simulink model "Non_Linearizzato_LQG"  (R2024b)
settings: Solver=VariableStepAuto  StartTime=0.0  StopTime=30  RelTol=1e-3
values from neighbouring files (symbols this model uses):
  Anom = A.NominalValue    [Parameter_CSI.m]
  Bnom = B.NominalValue    [Parameter_CSI.m]
  C = [(b_true*(Rp/L)^2-a_true*(Rp^2))*phi_dot*psi_dot*sin(psi)*cos(psi)+c_phi*phi_dot; -Ipz*(Rp/L)*phi_dot*psi_dot*cos(psi)+c_psi*psi_dot]    [Dinamica_CSI.m]    (also in Parameter_CSI.m = [1 0 0 0 0;0 0 1 0 0])
  D = append(d1,d1,tf(eye(2)),tf(eye(2)))    [D_K_controller2_FINAL.m]    (also in Parameter_CSI.m = zeros(2,2))
  G_tau_phi_nom_tf = minreal(tf(G_tau_phi_nom))    [Parameter_CSI.m]
  G_tau_psi_nom_tf = minreal(tf(G_tau_psi_nom))    [Parameter_CSI.m]
  Klqg = ss(Ac,-Bcy,Cc,-Dcy)    [LQG_controller_REG_FINAL.m]
  Rp_nom = 0.3    [Parameter_CSI.m]
  u_eq = [c_phi*vx/Rp_nom; 0]    [Parameter_CSI.m]
  vx = 1    [Dinamica_CSI.m]    (also in Parameter_CSI.m)
  x_eq = [0; 0; vx/Rp_nom; 0; 0]    [Parameter_CSI.m]
settings Model: Creator=alebe  LastModifiedBy=alebe

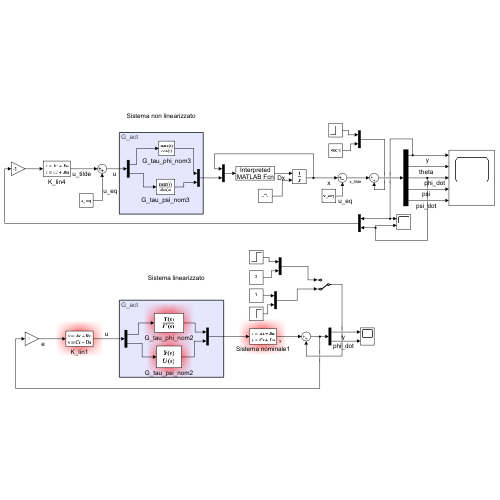
[thumbnail: Simulink's stored preview of the top-level diagram]
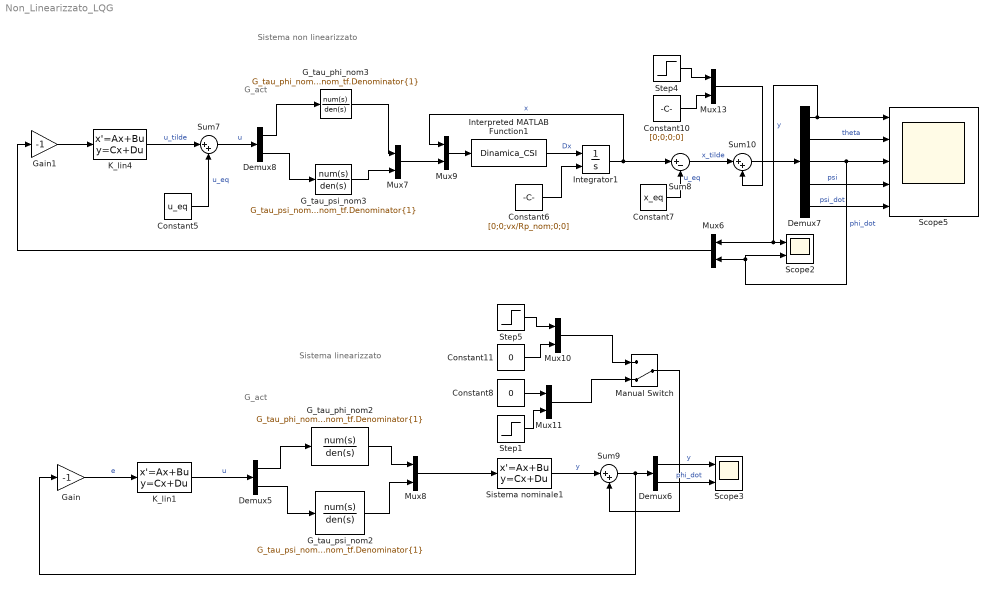
== system Non_Linearizzato_LQG ==
  note: G_act
  note: Sistema linearizzato
  note: G_act
  note: Sistema non linearizzato
  Constant10 : Constant  Value=[0;0;0;0]
  Constant11 : Constant  Value=0
  Constant5 : Constant  Value=u_eq
  Constant6 : Constant  Value=[0;0;vx/Rp_nom;0;0]
  Constant7 : Constant  Value=x_eq
  Constant8 : Constant  Value=0
  Demux5 : Demux  Outputs=2
  Demux6 : Demux  Outputs=2
  Demux7 : Demux  Outputs=5
  Demux8 : Demux  Outputs=2
  G_tau_phi_nom2 : TransferFcn  Numerator=G_tau_phi_nom_tf.Numerator{1}  Denominator=G_tau_phi_nom_tf.Denominator{1}
  G_tau_phi_nom3 : TransferFcn  Numerator=G_tau_phi_nom_tf.Numerator{1}  Denominator=G_tau_phi_nom_tf.Denominator{1}
  G_tau_psi_nom2 : TransferFcn  Numerator=G_tau_psi_nom_tf.Numerator{1}  Denominator=G_tau_psi_nom_tf.Denominator{1}
  G_tau_psi_nom3 : TransferFcn  Numerator=G_tau_psi_nom_tf.Numerator{1}  Denominator=G_tau_psi_nom_tf.Denominator{1}
  Gain : Gain  Gain=-1
  Gain1 : Gain  Gain=-1
  Integrator1 : Integrator  InitialConditionSource=external
  Interpreted MATLAB Function1 : MATLABFcn  MATLABFcn=Dinamica_CSI
  K_lin1 : StateSpace  A=Klqg.A  B=Klqg.B  C=Klqg.C  D=Klqg.D  InitialCondition=0
  K_lin4 : StateSpace  A=Klqg.A  B=Klqg.B  C=Klqg.C  D=Klqg.D  InitialCondition=0
  Manual Switch : ManualSwitch  CurrentSetting=0
  Mux{6..11,13} (7 alike) : Mux  Inputs=2
  Scope2 : Scope  NumInputPorts=2
  Scope3 : Scope  NumInputPorts=2
  Scope5 : Scope  NumInputPorts=5
  Sistema nominale1 : StateSpace  A=Anom  B=Bnom  C=C  D=D  InitialCondition=[0;0;0;0;0]
  Step1 : Step  SampleTime=0
  Step4 : Step  After=0.1  SampleTime=0
  Step5 : Step  After=0.1  SampleTime=0
  Sum10 : Sum  Inputs=|++
  Sum7 : Sum  Inputs=|++
  Sum8 : Sum  Inputs=|+-
  Sum9 : Sum  Inputs=|++
  wires:
  K_lin1/1 -> Demux5/1  "u"
  Gain/1 -> K_lin1/1  "e"
  Step4/1 -> Mux13/1
  Mux6/1 -> Gain1/1
  Demux6/1 -> Scope3/1  "y"
  Constant6/1 -> Integrator1/2
  Mux7/1 -> Mux9/2
  Demux7/3 -> Scope5/3, Scope2/2, Mux6/2  "phi_dot"
  G_tau_phi_nom2/1 -> Mux8/1
  G_tau_psi_nom2/1 -> Mux8/2
  G_tau_psi_nom3/1 -> Mux7/2
  Mux9/1 -> Interpreted MATLAB Function1/1
  Sum7/1 -> Demux8/1  "u"
  Demux6/2 -> Scope3/2  "phi_dot"
  Demux8/1 -> G_tau_phi_nom3/1
  Demux7/4 -> Scope5/4  "psi"
  Constant7/1 -> Sum8/2  "u_eq"
  Demux7/1 -> Mux6/1, Scope2/1, Scope5/1  "y"
  Constant5/1 -> Sum7/2  "u_eq"
  Demux7/5 -> Scope5/5  "psi_dot"
  Gain1/1 -> K_lin4/1
  Demux5/1 -> G_tau_phi_nom2/1
  K_lin4/1 -> Sum7/1  "u_tilde"
  Mux8/1 -> Sistema nominale1/1
  Sum8/1 -> Sum10/1  "x_tilde"
  Integrator1/1 -> Mux9/1, Sum8/1  "x"
  Sum10/1 -> Demux7/1
  Constant10/1 -> Mux13/2
  Demux8/2 -> G_tau_psi_nom3/1
  Sistema nominale1/1 -> Sum9/1  "y"
  Demux5/2 -> G_tau_psi_nom2/1
  Sum9/1 -> Gain/1, Demux6/1
  Mux10/1 -> Manual Switch/1
  Mux13/1 -> Sum10/2
  G_tau_phi_nom3/1 -> Mux7/1
  Constant11/1 -> Mux10/2
  Step5/1 -> Mux10/1
  Demux7/2 -> Scope5/2  "theta"
  Interpreted MATLAB Function1/1 -> Integrator1/1  "Dx"
  Step1/1 -> Mux11/2
  Constant8/1 -> Mux11/1
  Mux11/1 -> Manual Switch/2
  Manual Switch/1 -> Sum9/2
